simulink model "HMA_TB"  (R2020b)
settings: Solver=VariableStepAuto  StartTime=0.0  StopTime=100  RelTol=1e-3
PreLoadFcn:
  | N = 16
libraries: simulink x2, dspstat3 x2
settings Model: Creator=kschutz  LastModifiedBy=kschutz

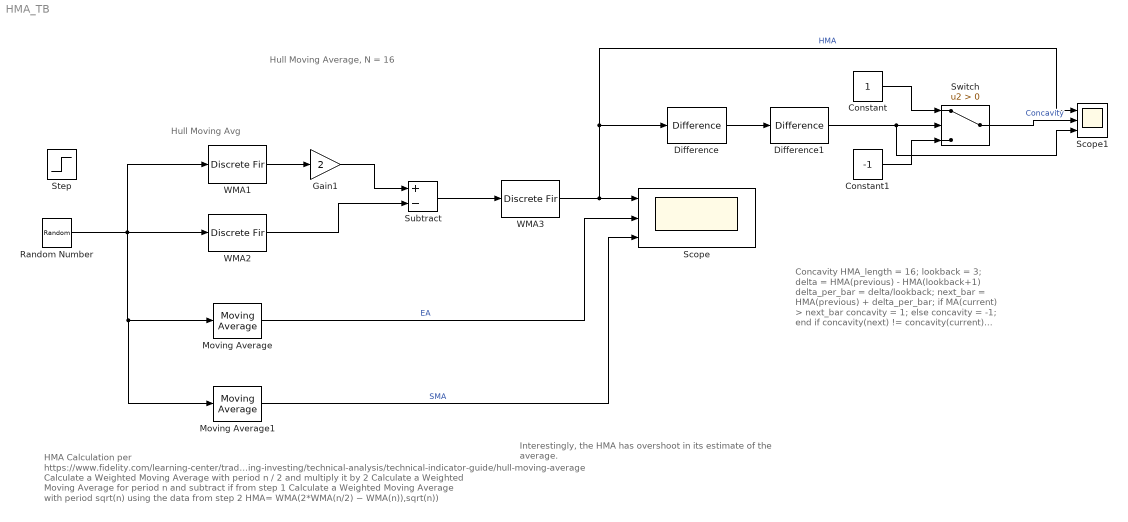
== system HMA_TB ==
  note: Concavity
      | HMA_length = 16;
      | lookback = 3;
      | delta = HMA(previous) - HMA(lookback+1)
      | delta_per_bar = delta/lookback;
      | next_bar = HMA(previous) + delta_per_bar;
      | if MA(current) > next_bar
      | 	concavity = 1;
      | else
      | 	concavity = -1;
      | end
      | if concavity(next) != concavity(current)
      | 	turning_point = HMA(current)
      | else
      |        turning_point = NaN;
      | end
      |
      | if turning_point and concavity == -1
      | 	buy = 1;
      | else
      | 	buy = NaN;
      | end
  note: Interestingly, the HMA has overshoot in its estimate of the
      | average.
  note: Hull Moving Avg
  note: HMA Calculation per
      |
      | https://www.fidelity.com/learning-center/trading-investing/technical-analysis/technical-indicator-guide/hull-moving-average
      |
      | Calculate a Weighted Moving Average with period n / 2 and multiply it by 2
      | Calculate a Weighted Moving Average for period n and subtract if from step 1
      | Calculate a Weighted Moving Average with period sqrt(n) using the data from step 2
      | HMA= WMA(2*WMA(n/2) − WMA(n)),sqrt(n))
  note: Hull Moving Average, N = 16
  Constant : Constant
  Constant1 : Constant  Value=-1
  Difference : simulink/Discrete/Difference  ICPrevInput=0.0  OutMin=[]  OutMax=[]  OutDataType=fixdt(1, 16)  OutScaling=2^-10  DoSatur=off
  Difference1 : simulink/Discrete/Difference  ICPrevInput=0.0  OutMin=[]  OutMax=[]  OutDataType=fixdt(1, 16)  OutScaling=2^-10  DoSatur=off
  Gain1 : Gain  Gain=2
  Moving Average : dspstat3/Moving Average  Method=Exponential weighting  ForgettingFactorPort=off  SpecifyWindowLength=on  WindowLength=20  ForgettingFactor=(N-1)/N  SimulateUsing=Interpreted execution
      settings: AttributesFormatString=FF = %<ForgettingFactor>
  Moving Average1 : dspstat3/Moving Average  Method=Sliding window  ForgettingFactorPort=off  SpecifyWindowLength=on  WindowLength=N  ForgettingFactor=15/16  SimulateUsing=Interpreted execution
      settings: AttributesFormatString=FF = %<ForgettingFactor>
  Random Number : RandomNumber  SampleTime=1
  Scope : Scope  NumInputPorts=3
  Scope1 : Scope  NumInputPorts=3
  Step : Step  After=10  SampleTime=1
  Subtract : Sum  Inputs=+-
  Switch : Switch  Criteria=u2 > Threshold
  WMA1 : DiscreteFir  Coefficients=[N/2:-1:1]/sum(1:N/2)
  WMA2 : DiscreteFir  Coefficients=[N:-1:1]/sum(1:N)
  WMA3 : DiscreteFir  Coefficients=[sqrt(N):-1:1]/sum(1:sqrt(N))
  wires:
  Random Number/1 -> WMA1/1, Moving Average1/1, Moving Average/1, WMA2/1
  WMA1/1 -> Gain1/1
  WMA2/1 -> Subtract/2
  Gain1/1 -> Subtract/1
  Subtract/1 -> WMA3/1
  WMA3/1 -> Scope1/1, Difference/1, Scope/1  "HMA"
  Moving Average/1 -> Scope/2  "EA"
  Moving Average1/1 -> Scope/3  "SMA"
  Difference/1 -> Difference1/1
  Difference1/1 -> Scope1/3, Switch/2
  Constant/1 -> Switch/1
  Constant1/1 -> Switch/3
  Switch/1 -> Scope1/2  "Concavity"
